simulink model "obserwator_kalmana"  (R2016b)
settings: Solver=FixedStepAuto  StartTime=0.0  StopTime=12  FixedStep=0.1  RelTol=1e-3  EnableMultiTasking=on
values from neighbouring files (symbols this model uses):
  A = [3 2 6 ... (first row only)    [obserwator_kalmana.m]    (also in por_odp.m)
  AK = A-HK*C    [obserwator_kalmana.m]    (also in por_odp.m)
  AL = A-HL*C    [obserwator_kalmana.m]    (also in por_odp.m)
  B = [1;1;0]    [obserwator_kalmana.m]    (also in por_odp.m)
  BK = [B-HK*D,HK]    [obserwator_kalmana.m]    (also in por_odp.m)
  BL = [B-HL*D,HL]    [obserwator_kalmana.m]    (also in por_odp.m)
  C = [0,1,1]    [obserwator_kalmana.m]    (also in por_odp.m)
  CK = C    [obserwator_kalmana.m]    (also in por_odp.m)
  CL = C    [obserwator_kalmana.m]    (also in por_odp.m)
  D = 0    [obserwator_kalmana.m]    (also in por_odp.m)
  DK = D    (= 0)    [obserwator_kalmana.m]    (also in por_odp.m)
  DL = D    (= 0)    [obserwator_kalmana.m]    (also in por_odp.m)
  HK = HK'    [obserwator_kalmana.m]    (also in por_odp.m)
  HL = HL'    [obserwator_kalmana.m]    (also in por_odp.m)
  Ki = K1(1,4)    [obserwator_kalmana.m]
  KK = K1(1,1:3)    [obserwator_kalmana.m]
  N = K*Nx+Nu    [obserwator_kalmana.m]
undefined symbols (not defined in the file or in its folder): K, sigbuilder_block
settings Model: Creator=student  LastModifiedBy=Admin
settings OptimizationCC: LifeSpan=inf
settings DebuggingCC: SFUnexpectedBacktrackingDiag=warning  SFNoUnconditionalDefaultTransitionDiag=warning  SFExecutionAtInitializationDiag=none
settings GRTTargetCC: TargetLangStandard=C89/C90 (ANSI)  GeneratePreprocessorConditionals=Disable all
settings ConfigComp: CovMetricSettings=dw  CovHtmlReporting=on  CovSaveCumulativeToWorkspaceVar=on  CovSaveSingleToWorkspaceVar=on  CovExternalEMLEnable=off

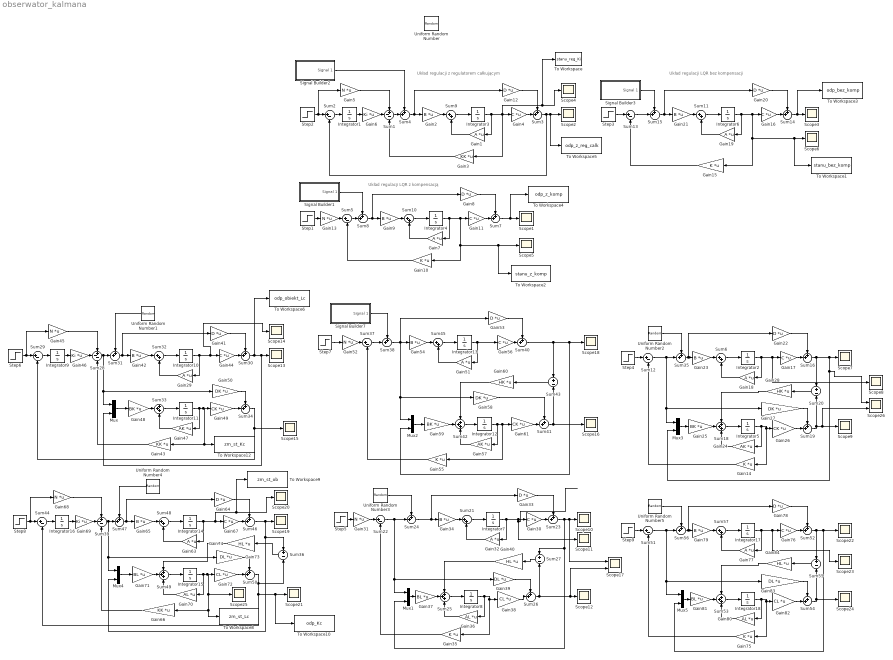
== system obserwator_kalmana ==
  note: Układ regulacji LQR z kompensacją
  note: Układ regulacji z regulatorem całkującym
  note: Układ regulacji LQR bez kompensacji
  Gain{1,7,18..19,29,32,51,63,77} (9 alike) : Gain  Gain=A  Multiplication=Matrix(K*u)
  Gain{10,14..15,35,55,75} (6 alike) : Gain  Gain=K  Multiplication=Matrix(K*u)
  Gain{4,11,16..17,30,44,56,67,76} (9 alike) : Gain  Gain=C  Multiplication=Matrix(K*u)
  Gain{8,12,20,22,33,41,53,64,78} (9 alike) : Gain  Gain=D  Multiplication=Matrix(K*u)
  Gain{5,13,31,45,52,68} (6 alike) : Gain  Gain=N  Multiplication=Matrix(K*u)
  Gain{2,9,21,23,34,42,54,65,79} (9 alike) : Gain  Gain=B  Multiplication=Matrix(K*u)
  Gain24 : Gain  Gain=AK  Multiplication=Matrix(K*u)
  Gain25 : Gain  Gain=BK  Multiplication=Matrix(K*u)
  Gain26 : Gain  Gain=CK  Multiplication=Matrix(K*u)
  Gain27 : Gain  Gain=DK  Multiplication=Matrix(K*u)
  Gain28 : Gain  Gain=HK  Multiplication=Matrix(K*u)
  Gain3 : Gain  Gain=KK  Multiplication=Matrix(K*u)
  Gain36 : Gain  Gain=AL  Multiplication=Matrix(K*u)
  Gain37 : Gain  Gain=BL  Multiplication=Matrix(K*u)
  Gain38 : Gain  Gain=CL  Multiplication=Matrix(K*u)
  Gain39 : Gain  Gain=DL  Multiplication=Matrix(K*u)
  Gain40 : Gain  Gain=HL  Multiplication=Matrix(K*u)
  Gain43 : Gain  Gain=KK  Multiplication=Matrix(K*u)
  Gain46 : Gain  Gain=Ki  Multiplication=Matrix(K*u)
  Gain47 : Gain  Gain=AK  Multiplication=Matrix(K*u)
  Gain48 : Gain  Gain=BK  Multiplication=Matrix(K*u)
  Gain49 : Gain  Gain=CK  Multiplication=Matrix(K*u)
  Gain50 : Gain  Gain=DK  Multiplication=Matrix(K*u)
  Gain57 : Gain  Gain=AK  Multiplication=Matrix(K*u)
  Gain58 : Gain  Gain=DK  Multiplication=Matrix(K*u)
  Gain59 : Gain  Gain=BK  Multiplication=Matrix(K*u)
  Gain6 : Gain  Gain=Ki  Multiplication=Matrix(K*u)
  Gain60 : Gain  Gain=HK  Multiplication=Matrix(K*u)
  Gain61 : Gain  Gain=CK  Multiplication=Matrix(K*u)
  Gain66 : Gain  Gain=KK  Multiplication=Matrix(K*u)
  Gain69 : Gain  Gain=Ki  Multiplication=Matrix(K*u)
  Gain70 : Gain  Gain=AL  Multiplication=Matrix(K*u)
  Gain71 : Gain  Gain=BL  Multiplication=Matrix(K*u)
  Gain72 : Gain  Gain=CL  Multiplication=Matrix(K*u)
  Gain73 : Gain  Gain=DL  Multiplication=Matrix(K*u)
  Gain74 : Gain  Gain=HL  Multiplication=Matrix(K*u)
  Gain80 : Gain  Gain=AL  Multiplication=Matrix(K*u)
  Gain81 : Gain  Gain=BL  Multiplication=Matrix(K*u)
  Gain82 : Gain  Gain=CL  Multiplication=Matrix(K*u)
  Gain83 : Gain  Gain=DL  Multiplication=Matrix(K*u)
  Gain84 : Gain  Gain=HL  Multiplication=Matrix(K*u)
  Integrator{1..18} (18 alike) : Integrator
  Mux{,1..5} (6 alike) : Mux  Inputs=2
  Scope{1..16,18..25} (24 alike) : Scope
  Scope17 : Scope  NumInputPorts=2
  Scope26 : Scope  NumInputPorts=2
  Signal Builder1 : Subsystem  Tag=STV Subsys  LoadFcn=sigbuilder_block('load');  StartFcn=sigbuilder_block('start');  StopFcn=sigbuilder_block('stop');  ClipboardFcn=sigbuilder_block('clipboard');  mask(Sigbuilder block){tuvar=[0:10]}
      mask help: Simulink:masks:SigbuilderBlock_MD
      mask init:
      | if ~strcmp(get_param(bdroot(gcbh),'SimulationStatus'),'stopped') tuvar = sigbuilder_block('maskInit'); end
      settings: CopyFcn=sigbuilder_block('copy');  DeleteFcn=sigbuilder_block('delete');  ModelCloseFcn=sigbuilder_block('modelClose');  PreSaveFcn=sigbuilder_block('preSave');  PauseFcn=sigbuilder_block('pause');  ContinueFcn=sigbuilder_block('continue');  NameChangeFcn=sigbuilder_block('namechange');  OpenFcn=sigbuilder_block('open',[437.6 199.2 550.4 400 ]);  CloseFcn=sigbuilder_block('close');
      mask Display: plot(0, 0, 100, 100,[2, 2, 32, 32, 2], [68, 8, 8, 68, 68],[32, 2], [38, 38], [32, 19, 2],[53, 60, 44], [32, 17, 17, 2],[16, 16, 31, 31]);txt = getActiveGroup(gcbh);text(2, 100, txt,'verticalAlignment', 'top');
  Signal Builder2 : Subsystem  Tag=STV Subsys  LoadFcn=sigbuilder_block('load');  StartFcn=sigbuilder_block('start');  StopFcn=sigbuilder_block('stop');  ClipboardFcn=sigbuilder_block('clipboard');  mask(Sigbuilder block){tuvar=[0:10]}
      mask help: Simulink:masks:SigbuilderBlock_MD
      mask init:
      | if ~strcmp(get_param(bdroot(gcbh),'SimulationStatus'),'stopped') tuvar = sigbuilder_block('maskInit'); end
      settings: CopyFcn=sigbuilder_block('copy');  DeleteFcn=sigbuilder_block('delete');  ModelCloseFcn=sigbuilder_block('modelClose');  PreSaveFcn=sigbuilder_block('preSave');  PauseFcn=sigbuilder_block('pause');  ContinueFcn=sigbuilder_block('continue');  NameChangeFcn=sigbuilder_block('namechange');  OpenFcn=sigbuilder_block('open',[437.25 153.75 550.5 359.25 ]);  CloseFcn=sigbuilder_block('close');
      mask Display: plot(0, 0, 100, 100,[2, 2, 32, 32, 2], [68, 8, 8, 68, 68],[32, 2], [38, 38], [32, 19, 2],[53, 60, 44], [32, 17, 17, 2],[16, 16, 31, 31]);txt = getActiveGroup(gcbh);text(2, 100, txt,'verticalAlignment', 'top');
  Signal Builder3 : Subsystem  Tag=STV Subsys  LoadFcn=sigbuilder_block('load');  StartFcn=sigbuilder_block('start');  StopFcn=sigbuilder_block('stop');  ClipboardFcn=sigbuilder_block('clipboard');  mask(Sigbuilder block){tuvar=[0:10]}
      mask help: Simulink:masks:SigbuilderBlock_MD
      mask init:
      | if ~strcmp(get_param(bdroot(gcbh),'SimulationStatus'),'stopped') tuvar = sigbuilder_block('maskInit'); end
      settings: CopyFcn=sigbuilder_block('copy');  DeleteFcn=sigbuilder_block('delete');  ModelCloseFcn=sigbuilder_block('modelClose');  PreSaveFcn=sigbuilder_block('preSave');  PauseFcn=sigbuilder_block('pause');  ContinueFcn=sigbuilder_block('continue');  NameChangeFcn=sigbuilder_block('namechange');  OpenFcn=sigbuilder_block('open',[437.25 153.75 550.5 359.25 ]);  CloseFcn=sigbuilder_block('close');
      mask Display: plot(0, 0, 100, 100,[2, 2, 32, 32, 2], [68, 8, 8, 68, 68],[32, 2], [38, 38], [32, 19, 2],[53, 60, 44], [32, 17, 17, 2],[16, 16, 31, 31]);txt = getActiveGroup(gcbh);text(2, 100, txt,'verticalAlignment', 'top');
  Signal Builder7 : Subsystem  Tag=STV Subsys  LoadFcn=sigbuilder_block('load');  StartFcn=sigbuilder_block('start');  StopFcn=sigbuilder_block('stop');  ClipboardFcn=sigbuilder_block('clipboard');  mask(Sigbuilder block){tuvar=[0:10]}
      mask help: Simulink:masks:SigbuilderBlock_MD
      mask init:
      | if ~strcmp(get_param(bdroot(gcbh),'SimulationStatus'),'stopped') tuvar = sigbuilder_block('maskInit'); end
      settings: CopyFcn=sigbuilder_block('copy');  DeleteFcn=sigbuilder_block('delete');  ModelCloseFcn=sigbuilder_block('modelClose');  PreSaveFcn=sigbuilder_block('preSave');  PauseFcn=sigbuilder_block('pause');  ContinueFcn=sigbuilder_block('continue');  NameChangeFcn=sigbuilder_block('namechange');  OpenFcn=sigbuilder_block('open',[437.6 199.2 550.4 400 ]);  CloseFcn=sigbuilder_block('close');
      mask Display: plot(0, 0, 100, 100,[2, 2, 32, 32, 2], [68, 8, 8, 68, 68],[32, 2], [38, 38], [32, 19, 2],[53, 60, 44], [32, 17, 17, 2],[16, 16, 31, 31]);txt = getActiveGroup(gcbh);text(2, 100, txt,'verticalAlignment', 'top');
  Step{1..3,5..8} (7 alike) : Step  Time=0  SampleTime=0
  Step4 : Step  SampleTime=0
  Step9 : Step  SampleTime=0
  Sum1 : Sum  Inputs=+--
  Sum{6,9..11,21,32,45,48,57} (9 alike) : Sum  Inputs=|++
  Sum{2,5,12..13,22,29,37,44,51} (9 alike) : Sum  Inputs=|+-
  Sum{3..4,7..8,14..16,19,23..24,26,30..31,34..35,38,40..41,46..47,50,52,54,56} (24 alike) : Sum  Inputs=++|
  Sum{18,25,33,42,49,53} (6 alike) : Sum  Inputs=+++
  Sum{20,27,36,55} (4 alike) : Sum  Inputs=+-
  Sum28 : Sum  Inputs=+--
  Sum39 : Sum  Inputs=+--
  Sum43 : Sum  Inputs=+|-
  To Workspace : ToWorkspace  VariableName=stanu_reg_Ki  SaveFormat=Timeseries  SampleTime=-1
  To Workspace1 : ToWorkspace  VariableName=stanu_bez_komp  SaveFormat=Timeseries  SampleTime=-1
  To Workspace10 : ToWorkspace  VariableName=odp_Kc  SaveFormat=Timeseries  SampleTime=-1
  To Workspace12 : ToWorkspace  VariableName=zm_st_Kc  SaveFormat=Timeseries  SampleTime=-1
  To Workspace2 : ToWorkspace  VariableName=stanu_z_komp  SaveFormat=Timeseries  SampleTime=-1
  To Workspace3 : ToWorkspace  VariableName=odp_bez_komp  SaveFormat=Timeseries  SampleTime=-1
  To Workspace4 : ToWorkspace  VariableName=odp_z_komp  SaveFormat=Timeseries  SampleTime=-1
  To Workspace5 : ToWorkspace  VariableName=odp_z_reg_calk  SaveFormat=Timeseries  SampleTime=-1
  To Workspace6 : ToWorkspace  VariableName=odp_obiekt_Lc  SaveFormat=Timeseries  SampleTime=-1
  To Workspace8 : ToWorkspace  VariableName=zm_st_Lc  SaveFormat=Timeseries  SampleTime=-1
  To Workspace9 : ToWorkspace  VariableName=zm_st_ob  SaveFormat=Timeseries  SampleTime=-1
  Uniform Random Number : UniformRandomNumber  SampleTime=1
  Uniform Random Number{1..5} (5 alike) : UniformRandomNumber  SampleTime=0.1
  wires:
  Sum3/1 -> To Workspace5/1, Scope2/1, Sum2/2
  Integrator3/1 -> Gain1/1, Gain3/1, To Workspace/1, Scope4/1, Gain4/1
  Step2/1 -> Gain5/1, Sum2/1
  Gain12/1 -> Sum3/1
  Gain4/1 -> Sum3/2
  Sum9/1 -> Integrator3/1
  Gain1/1 -> Sum9/2
  Gain2/1 -> Sum9/1
  Sum1/1 -> Sum4/2
  Sum2/1 -> Integrator1/1
  Integrator1/1 -> Gain6/1
  Gain6/1 -> Sum1/2
  Gain3/1 -> Sum1/3
  Gain5/1 -> Sum1/1
  Sum7/1 -> To Workspace4/1, Scope1/1
  Integrator4/1 -> To Workspace2/1, Scope5/1, Gain10/1, Gain11/1, Gain7/1
  Gain8/1 -> Sum7/1
  Gain11/1 -> Sum7/2
  Sum10/1 -> Integrator4/1
  Gain7/1 -> Sum10/2
  Gain9/1 -> Sum10/1
  Sum5/1 -> Sum8/2
  Step1/1 -> Gain13/1
  Gain13/1 -> Sum5/1
  Gain10/1 -> Sum5/2
  Signal Builder1/1(Signal 1) -> Sum8/1
  Sum14/1 -> To Workspace3/1, Scope3/1
  Integrator6/1 -> Gain19/1, Gain16/1, To Workspace1/1, Scope6/1, Gain15/1
  Step3/1 -> Sum13/1
  Gain20/1 -> Sum14/1
  Gain16/1 -> Sum14/2
  Sum11/1 -> Integrator6/1
  Gain19/1 -> Sum11/2
  Gain21/1 -> Sum11/1
  Sum13/1 -> Sum15/2
  Signal Builder3/1(Signal 1) -> Sum15/1
  Gain15/1 -> Sum13/2
  Integrator2/1 -> Scope8/1, Gain17/1, Gain18/1
  Step4/1 -> Sum12/1
  Gain22/1 -> Sum16/1
  Gain17/1 -> Sum16/2
  Sum6/1 -> Integrator2/1
  Gain18/1 -> Sum6/2
  Gain23/1 -> Sum6/1
  Gain14/1 -> Sum12/2
  Integrator5/1 -> Gain14/1, Gain26/1, Gain24/1
  Sum18/1 -> Integrator5/1
  Gain27/1 -> Sum19/1
  Gain26/1 -> Sum19/2
  Sum19/1 -> Scope26/2, Scope9/1, Sum20/2
  Gain25/1 -> Sum18/2
  Gain24/1 -> Sum18/3
  Sum20/1 -> Gain28/1
  Gain28/1 -> Sum18/1
  Sum23/1 -> Mux1/2, Sum27/1, Scope17/1, Scope10/1
  Integrator7/1 -> Gain32/1, Gain30/1, Scope11/1
  Gain33/1 -> Sum23/1
  Gain30/1 -> Sum23/2
  Sum21/1 -> Integrator7/1
  Gain32/1 -> Sum21/2
  Gain34/1 -> Sum21/1
  Gain35/1 -> Sum22/2
  Integrator8/1 -> Gain36/1, Gain38/1, Gain35/1
  Sum25/1 -> Integrator8/1
  Gain39/1 -> Sum26/1
  Gain38/1 -> Sum26/2
  Sum26/1 -> Sum27/2, Scope17/2, Scope12/1
  Gain37/1 -> Sum25/2
  Gain36/1 -> Sum25/3
  Sum27/1 -> Gain40/1
  Gain40/1 -> Sum25/1
  Sum30/1 -> To Workspace6/1, Mux/2, Scope13/1
  Integrator10/1 -> Scope14/1, Gain44/1, Gain29/1
  Step6/1 -> Sum29/1, Gain45/1
  Gain41/1 -> Sum30/1
  Gain44/1 -> Sum30/2
  Sum32/1 -> Integrator10/1
  Gain29/1 -> Sum32/2
  Gain42/1 -> Sum32/1
  Sum29/1 -> Integrator9/1
  Integrator9/1 -> Gain46/1
  Gain46/1 -> Sum28/2
  Gain43/1 -> Sum28/3
  Gain45/1 -> Sum28/1
  Sum28/1 -> Gain50/1, Mux/1, Sum31/2
  Uniform Random Number1/1 -> Sum31/1
  Sum31/1 -> Gain42/1, Gain41/1
  Integrator11/1 -> Gain47/1, Gain43/1, To Workspace12/1, Gain49/1
  Sum33/1 -> Integrator11/1
  Gain50/1 -> Sum34/1
  Gain49/1 -> Sum34/2
  Sum34/1 -> Sum29/2, Scope15/1
  Gain48/1 -> Sum33/2
  Gain47/1 -> Sum33/3
  Mux/1 -> Gain48/1
  Sum35/1 -> Gain22/1, Gain23/1
  Uniform Random Number2/1 -> Sum35/1
  Sum24/1 -> Gain33/1, Gain34/1
  Sum15/1 -> Gain20/1, Gain21/1
  Sum4/1 -> Gain12/1, Gain2/1
  Sum8/1 -> Gain8/1, Gain9/1
  Signal Builder2/1(Signal 1) -> Sum4/1
  Gain55/1 -> Sum37/2
  Sum40/1 -> Sum43/1, Mux2/2, Scope18/1
  Gain53/1 -> Sum40/1
  Gain56/1 -> Sum40/2
  Sum45/1 -> Integrator13/1
  Gain51/1 -> Sum45/2
  Gain54/1 -> Sum45/1
  Sum38/1 -> Gain58/1, Mux2/1, Gain54/1, Gain53/1
  Sum41/1 -> Sum43/2, Scope16/1
  Gain58/1 -> Sum41/1
  Gain61/1 -> Sum41/2
  Sum42/1 -> Integrator12/1
  Gain59/1 -> Sum42/2
  Gain57/1 -> Sum42/3
  Gain60/1 -> Sum42/1
  Sum43/1 -> Gain60/1
  Gain52/1 -> Sum37/1
  Step7/1 -> Gain52/1
  Integrator12/1 -> Gain55/1, Gain61/1, Gain57/1
  Integrator13/1 -> Gain51/1, Gain56/1
  Sum37/1 -> Sum38/2
  Signal Builder7/1(Signal 1) -> Sum38/1
  Mux1/1 -> Gain37/1
  Mux2/1 -> Gain59/1
  Step5/1 -> Gain31/1
  Gain31/1 -> Sum22/1
  Uniform Random Number3/1 -> Sum24/1
  Sum22/1 -> Gain39/1, Mux1/1, Sum24/2
  Sum46/1 -> Sum36/1, Mux4/2, Scope19/1
  Integrator14/1 -> Gain67/1, To Workspace9/1, Scope20/1, Gain63/1
  Step8/1 -> Sum44/1, Gain68/1
  Gain64/1 -> Sum46/1
  Gain67/1 -> Sum46/2
  Sum48/1 -> Integrator14/1
  Gain63/1 -> Sum48/2
  Gain65/1 -> Sum48/1
  Sum44/1 -> Integrator16/1
  Integrator16/1 -> Gain69/1
  Gain69/1 -> Sum39/2
  Gain66/1 -> Sum39/3
  Gain68/1 -> Sum39/1
  Sum39/1 -> Gain73/1, Mux4/1, Sum47/2
  Uniform Random Number4/1 -> Sum47/1
  Sum47/1 -> Gain65/1, Gain64/1
  Sum49/1 -> Integrator15/1
  Gain73/1 -> Sum50/1
  Gain72/1 -> Sum50/2
  Sum50/1 -> Sum36/2, Sum44/2, To Workspace10/1, Scope21/1
  Gain71/1 -> Sum49/2
  Gain70/1 -> Sum49/3
  Mux4/1 -> Gain71/1
  Sum36/1 -> Gain74/1
  Gain74/1 -> Sum49/1
  Sum52/1 -> Sum55/1, Mux5/2, Scope22/1
  Integrator17/1 -> Scope23/1, Gain76/1, Gain77/1
  Step9/1 -> Sum51/1
  Gain78/1 -> Sum52/1
  Gain76/1 -> Sum52/2
  Sum57/1 -> Integrator17/1
  Gain77/1 -> Sum57/2
  Gain79/1 -> Sum57/1
  Sum51/1 -> Sum56/2, Gain83/1, Mux5/1
  Gain75/1 -> Sum51/2
  Integrator18/1 -> Gain75/1, Gain82/1, Gain80/1
  Sum53/1 -> Integrator18/1
  Gain83/1 -> Sum54/1
  Gain82/1 -> Sum54/2
  Sum54/1 -> Scope24/1, Sum55/2
  Gain81/1 -> Sum53/2
  Gain80/1 -> Sum53/3
  Sum55/1 -> Gain84/1
  Gain84/1 -> Sum53/1
  Sum56/1 -> Gain78/1, Gain79/1
  Uniform Random Number5/1 -> Sum56/1
  Mux5/1 -> Gain81/1
  Integrator15/1 -> Gain70/1, Scope25/1, To Workspace8/1, Gain66/1, Gain72/1
  Sum12/1 -> Sum35/2, Mux3/1, Gain27/1
  Mux3/1 -> Gain25/1
  Sum16/1 -> Sum20/1, Scope7/1, Scope26/1, Mux3/2

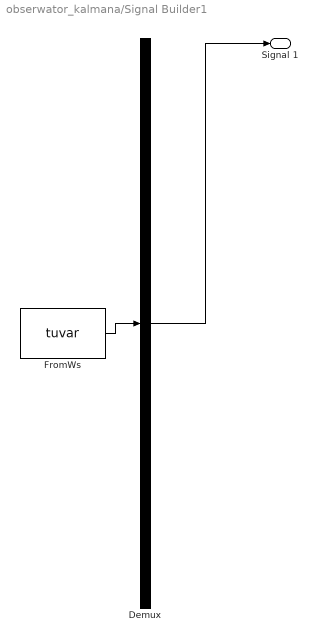
== system obserwator_kalmana/Signal Builder1 ==
  Demux : Demux  Tag=STV Demux  Outputs=1
  FromWs : FromWorkspace  Tag=STV FromWs  VariableName=tuvar  SampleTime=0
      SigBuilderData=|
      | common.afterFinalStr = 'Extrapolate'
      | common.sampleTime = 0
      | dataSet.timeRange = [0 10]
      | dataSet.name = 'Group 1'
      | sbobj.Groups.Name = 'Group 1'
      | sbobj.Groups.Signals.Name = 'Signal 1'
      | sbobj.Groups.Signals.XData = [0 4 4 5 5 10]
      | sbobj.Groups.Signals.YData = [0 0 1 1 0 0]
  Signal 1 : Outport  Tag=STV Outport
  wires:
  Demux/1 -> Signal 1/1
  FromWs/1 -> Demux/1

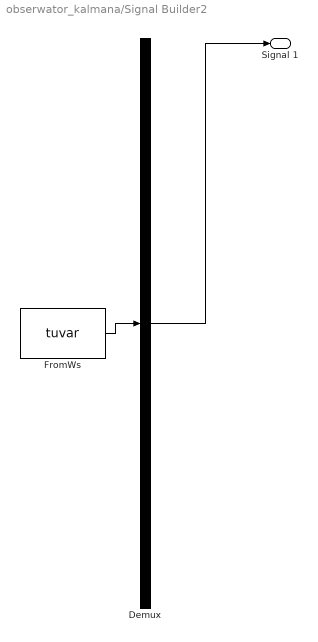
== system obserwator_kalmana/Signal Builder2 ==
  Demux : Demux  Tag=STV Demux  Outputs=1
  FromWs : FromWorkspace  Tag=STV FromWs  VariableName=tuvar  SampleTime=0
      SigBuilderData=|
      | common.afterFinalStr = 'Extrapolate'
      | common.sampleTime = 0
      | dataSet.timeRange = [0 10]
      | dataSet.name = 'Group 1'
      | sbobj.Groups.Name = 'Group 1'
      | sbobj.Groups.Signals.Name = 'Signal 1'
      | sbobj.Groups.Signals.XData = [0 4 4 5 5 10]
      | sbobj.Groups.Signals.YData = [0 0 1 1 0 0]
  Signal 1 : Outport  Tag=STV Outport
  wires:
  FromWs/1 -> Demux/1
  Demux/1 -> Signal 1/1

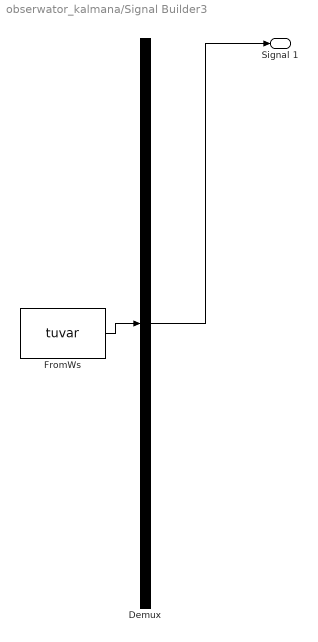
== system obserwator_kalmana/Signal Builder3 ==
  Demux : Demux  Tag=STV Demux  Outputs=1
  FromWs : FromWorkspace  Tag=STV FromWs  VariableName=tuvar  SampleTime=0
      SigBuilderData=|
      | common.afterFinalStr = 'Extrapolate'
      | common.sampleTime = 0
      | dataSet.timeRange = [0 10]
      | dataSet.name = 'Group 1'
      | sbobj.Groups.Name = 'Group 1'
      | sbobj.Groups.Signals.Name = 'Signal 1'
      | sbobj.Groups.Signals.XData = [0 4 4 5 5 10]
      | sbobj.Groups.Signals.YData = [0 0 1 1 0 0]
  Signal 1 : Outport  Tag=STV Outport
  wires:
  FromWs/1 -> Demux/1
  Demux/1 -> Signal 1/1

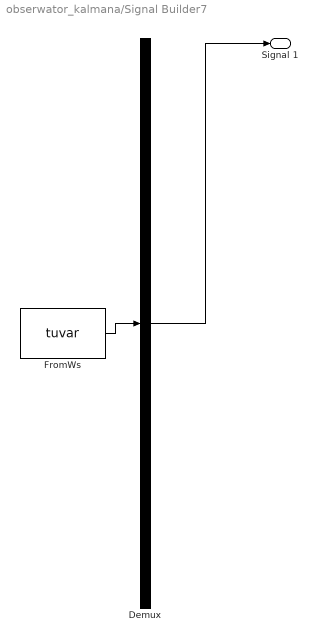
== system obserwator_kalmana/Signal Builder7 ==
  Demux : Demux  Tag=STV Demux  Outputs=1
  FromWs : FromWorkspace  Tag=STV FromWs  VariableName=tuvar  SampleTime=0
      SigBuilderData=|
      | common.afterFinalStr = 'Extrapolate'
      | common.sampleTime = 0
      | dataSet.timeRange = [0 10]
      | dataSet.name = 'Group 1'
      | sbobj.Groups.Name = 'Group 1'
      | sbobj.Groups.Signals.Name = 'Signal 1'
      | sbobj.Groups.Signals.XData = [0 4 4 5 5 10]
      | sbobj.Groups.Signals.YData = [0 0 1 1 0 0]
  Signal 1 : Outport  Tag=STV Outport
  wires:
  FromWs/1 -> Demux/1
  Demux/1 -> Signal 1/1
